simulink model "qsg_4sf"  (R2019a)
settings: Solver=VariableStepAuto  StartTime=0.0  StopTime=10.0  RelTol=1e-3
libraries: Solver_SF x4
settings Model: Creator=jhu  LastModifiedBy=asun
settings DebuggingCC: UnconnectedInputMsg=none  UnconnectedOutputMsg=none  UnconnectedLineMsg=none  SFMachineParentedDataDiag=error  ArithmeticOperatorsInVariantConditions=warning

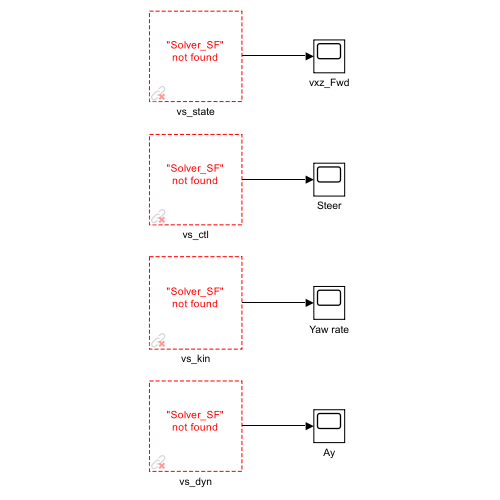
[thumbnail: Simulink's stored preview of the top-level diagram]
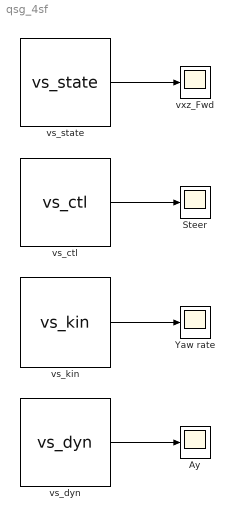
== system qsg_4sf ==
  Ay : Scope
  Steer : Scope
  Yaw rate : Scope
  vs_ctl : Solver_SF/CarSim Multi-Wrappers/vs_ctl  Priority=2  SIMFILE=simfile.sim
  vs_dyn : Solver_SF/CarSim Multi-Wrappers/vs_dyn  Priority=4  SIMFILE=simfile.sim
  vs_kin : Solver_SF/CarSim Multi-Wrappers/vs_kin  Priority=3  SIMFILE=simfile.sim
  vs_state : Solver_SF/CarSim Multi-Wrappers/vs_state  Priority=1  SIMFILE=simfile.sim
  vxz_Fwd : Scope
  wires:
  vs_ctl/1 -> Steer/1
  vs_dyn/1 -> Ay/1
  vs_kin/1 -> Yaw rate/1
  vs_state/1 -> vxz_Fwd/1
